simulink model "matrice_gravite"  (R2022b)
settings: Solver=VariableStepAuto  StartTime=0.0  StopTime=2  RelTol=1e-3
InitFcn:
  | l1=0.6;
  | l2=0.3;
  | m1=1;
  | m2=0.5;
settings Model: Creator=cheye  LastModifiedBy=cheye

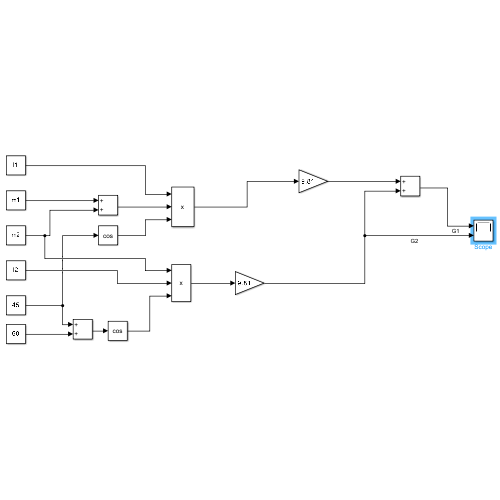
[thumbnail: Simulink's stored preview of the top-level diagram]
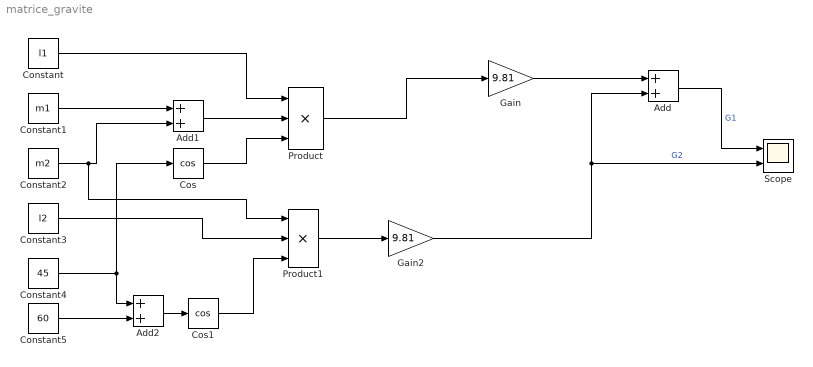
== system matrice_gravite ==
  Add : Sum
  Add1 : Sum
  Add2 : Sum
  Constant : Constant  Value=l1
  Constant1 : Constant  Value=m1
  Constant2 : Constant  Value=m2
  Constant3 : Constant  Value=l2
  Constant4 : Constant  Value=45
  Constant5 : Constant  Value=60
  Cos : Trigonometry  Operator=cos
  Cos1 : Trigonometry  Operator=cos
  Gain : Gain  Gain=9.81
  Gain2 : Gain  Gain=9.81
  Product : Product  Inputs=3
  Product1 : Product  Inputs=3
  Scope : Scope  NumInputPorts=2
  wires:
  Constant4/1 -> Cos/1, Add2/1
  Constant1/1 -> Add1/1
  Constant2/1 -> Product1/1, Add1/2
  Cos/1 -> Product/3
  Add1/1 -> Product/2
  Constant/1 -> Product/1
  Product/1 -> Gain/1
  Gain/1 -> Add/1
  Add/1 -> Scope/1  "G1"
  Constant3/1 -> Product1/2
  Constant5/1 -> Add2/2
  Add2/1 -> Cos1/1
  Cos1/1 -> Product1/3
  Product1/1 -> Gain2/1
  Gain2/1 -> Scope/2, Add/2  "G2"
